simulink model "Ecuaciones_Fisicas_2020a"  (Simulink 10.1)
settings: Solver=FixedStepAuto  StartTime=0.0  StopTime=5  FixedStep=0.001  RelTol=1e-3
undefined symbols (not defined in the file or in its folder): magnitude, sigbuilder_block
libraries: simulink x2, simulink_extras x1
settings Model: Creator=alvar  LastModifiedBy=alvar  PauseTimes=2.78
settings DataIOCC: SaveFormat=Dataset  ReturnWorkspaceOutputs=on
settings OptimizationCC: LifeSpan=auto
settings DebuggingCC: UnderspecifiedInitializationDetection=Simplified  MergeDetectMultiDrivingBlocksExec=error  SFUnexpectedBacktrackingDiag=error  SFNoUnconditionalDefaultTransitionDiag=error  SFExecutionAtInitializationDiag=warning  ArithmeticOperatorsInVariantConditions=error
settings HardwareCC: ProdBitPerPointer=64  ProdBitPerSizeT=64  ProdBitPerPtrDiffT=64  ProdLargestAtomicFloat=Float  ProdIntDivRoundTo=Zero  ProdEndianess=LittleEndian  ProdWordSize=64  ProdHWDeviceType=Intel->x86-64 (Windows64)
settings ModelReferenceCC: PropagateSignalLabelsOutOfModel=on
settings SFSimCC: SimUseLocalCustomCode=on  CustomCodeUndefinedFunction=FilterOut
settings RTWCC: RTWUseLocalCustomCode=on
settings CodeAppCC: StateflowObjectComments=off
settings GRTTargetCC: TargetLangStandard=C99 (ISO)  CombineOutputUpdateFcns=on  GRTInterface=off
settings ConfigComp: CovMetricSettings=dwe  CovSaveCumulativeToWorkspaceVar=off  CovSaveSingleToWorkspaceVar=off  CovExternalEMLEnable=on

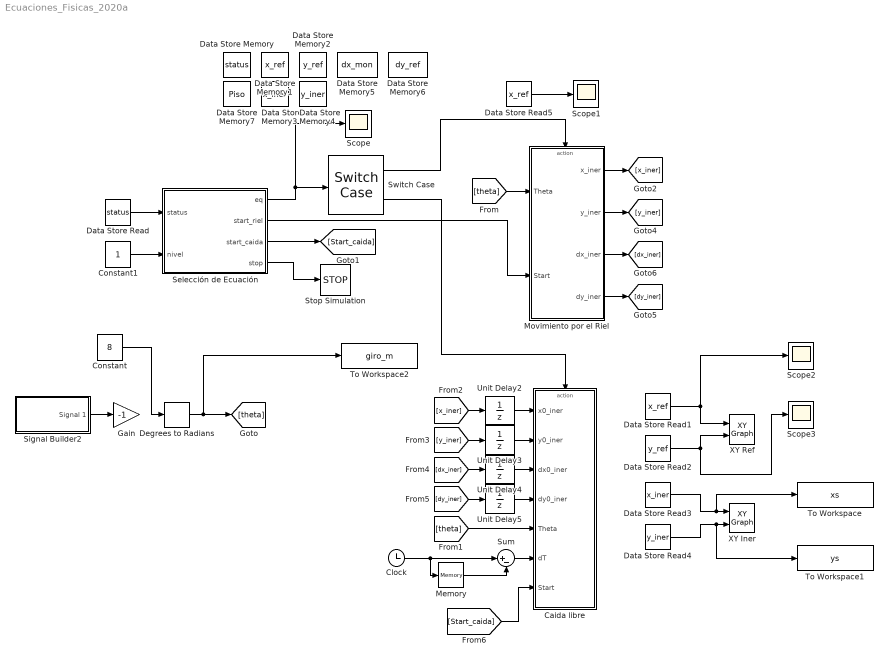
== system Ecuaciones_Fisicas_2020a ==
  Caida libre : Subsystem  TreatAsAtomicUnit=on
  Clock : Clock
  Constant : Constant  Value=8
  Constant1 : Constant
  Data Store Memory : DataStoreMemory  DataStoreName=status  ReadBeforeWriteMsg=warning  WriteAfterWriteMsg=warning  WriteAfterReadMsg=warning  ShowAdditionalParam=off  OutDataTypeStr=double
  Data Store Memory1 : DataStoreMemory  DataStoreName=x_ref  ReadBeforeWriteMsg=warning  WriteAfterWriteMsg=warning  WriteAfterReadMsg=warning  InitialValue=-0.11  ShowAdditionalParam=off  OutDataTypeStr=double
  Data Store Memory2 : DataStoreMemory  DataStoreName=y_ref  ReadBeforeWriteMsg=warning  WriteAfterWriteMsg=warning  WriteAfterReadMsg=warning  ShowAdditionalParam=off  OutDataTypeStr=double
  Data Store Memory3 : DataStoreMemory  DataStoreName=x_iner  ReadBeforeWriteMsg=warning  WriteAfterWriteMsg=warning  WriteAfterReadMsg=warning  InitialValue=-0.11  ShowAdditionalParam=off  OutDataTypeStr=double
  Data Store Memory4 : DataStoreMemory  DataStoreName=y_iner  ReadBeforeWriteMsg=warning  WriteAfterWriteMsg=warning  WriteAfterReadMsg=warning  ShowAdditionalParam=off  OutDataTypeStr=double
  Data Store Memory5 : DataStoreMemory  DataStoreName=dx_mon  ReadBeforeWriteMsg=warning  WriteAfterWriteMsg=warning  WriteAfterReadMsg=warning  ShowAdditionalParam=off  OutDataTypeStr=double
  Data Store Memory6 : DataStoreMemory  DataStoreName=dy_ref  ReadBeforeWriteMsg=warning  WriteAfterWriteMsg=warning  WriteAfterReadMsg=warning  ShowAdditionalParam=off  OutDataTypeStr=double
  Data Store Memory7 : DataStoreMemory  DataStoreName=Piso  ReadBeforeWriteMsg=warning  WriteAfterWriteMsg=warning  WriteAfterReadMsg=warning  InitialValue=1  ShowAdditionalParam=off  OutDataTypeStr=double
  Data Store Read : DataStoreRead  DataStoreName=status
  Data Store Read1 : DataStoreRead  DataStoreName=x_ref
  Data Store Read2 : DataStoreRead  DataStoreName=y_ref
  Data Store Read3 : DataStoreRead  DataStoreName=x_iner
  Data Store Read4 : DataStoreRead  DataStoreName=y_iner
  Data Store Read5 : DataStoreRead  DataStoreName=x_ref
  Degrees to Radians : simulink_extras/Transformations/Degrees to Radians
  Gain : Gain  Gain=-1
  Memory : Memory
  Movimiento por el Riel : Subsystem  TreatAsAtomicUnit=on
  Scope{,1..3} (4 alike) : Scope
  Selección de Ecuación : MATLAB Function  TreatAsAtomicUnit=on
  Signal Builder2 : Subsystem  Tag=STV Subsys  LoadFcn=sigbuilder_block('load');  StartFcn=sigbuilder_block('start');  StopFcn=sigbuilder_block('stop');  ClipboardFcn=sigbuilder_block('clipboard');  mask(Sigbuilder block){tuvar=[0:10]}
      mask help: Simulink:masks:SigbuilderBlock_MD
      mask init:
      | if ~strcmp(get_param(bdroot(gcbh),'SimulationStatus'),'stopped') tuvar = sigbuilder_block('maskInit'); end
      settings: CopyFcn=sigbuilder_block('copy');  DeleteFcn=sigbuilder_block('delete');  ModelCloseFcn=sigbuilder_block('modelClose');  PreSaveFcn=sigbuilder_block('preSave');  PauseFcn=sigbuilder_block('pause');  ContinueFcn=sigbuilder_block('continue');  NameChangeFcn=sigbuilder_block('namechange');  OpenFcn=sigbuilder_block('open',[516 235.5 550.5 399.75 ]);  CloseFcn=sigbuilder_block('close');
      mask Display: plot(0, 0, 100, 100,[2, 2, 32, 32, 2], [68, 8, 8, 68, 68],[32, 2], [38, 38], [32, 19, 2],[53, 60, 44], [32, 17, 17, 2],[16, 16, 31, 31]);txt = getActiveGroup(gcbh);text(2, 100, txt,'verticalAlignment', 'top');
  Stop Simulation : Stop
  Sum : Sum  Inputs=|+-
  Switch Case : SwitchCase  CaseConditions={1,2}  ShowDefaultCase=off
  To Workspace : ToWorkspace  VariableName=xs  SampleTime=0.01
  To Workspace1 : ToWorkspace  VariableName=ys  SampleTime=0.01
  To Workspace2 : ToWorkspace  VariableName=giro_m  SampleTime=0.01
  Unit Delay{2..5} (4 alike) : UnitDelay  SampleTime=-1  HasFrameUpgradeWarning=on
  XY Iner : simulink/Sinks/XY Graph  xmin=-0.15  xmax=0.15  ymin=-0.3  ymax=0.2  st=-1
  XY Ref : simulink/Sinks/XY Graph  xmin=-0.15  xmax=0.15  ymin=-0.3  ymax=0.2  st=-1
  wires:
  Switch Case/1 -> Movimiento por el Riel/Action
  [theta] -> Movimiento por el Riel/1(Theta)
  Switch Case/2 -> Caida libre/Action
  Selección de Ecuación/1(eq) -> Switch Case/1, Scope/1
  Data Store Read/1 -> Selección de Ecuación/1(status)
  Degrees to Radians/1 -> To Workspace2/1, [theta]
  Memory/1 -> Sum/2
  Clock/1 -> Sum/1, Memory/1
  Sum/1 -> Caida libre/6(dT)
  [x_iner] -> Unit Delay2/1
  Unit Delay2/1 -> Caida libre/1(x0_iner)
  [y_iner] -> Unit Delay3/1
  Unit Delay3/1 -> Caida libre/2(y0_iner)
  [dx_iner] -> Unit Delay4/1
  Unit Delay4/1 -> Caida libre/3(dx0_iner)
  [dy_iner] -> Unit Delay5/1
  Unit Delay5/1 -> Caida libre/4(dy0_iner)
  [theta] -> Caida libre/5(Theta)
  Data Store Read1/1 -> Scope2/1, XY Ref/1
  Data Store Read2/1 -> XY Ref/2, Scope3/1
  Data Store Read4/1 -> To Workspace1/1, XY Iner/2
  Data Store Read3/1 -> To Workspace/1, XY Iner/1
  Movimiento por el Riel/1(x_iner) -> [x_iner]
  Movimiento por el Riel/3(dx_iner) -> [dx_iner]
  Movimiento por el Riel/2(y_iner) -> [y_iner]
  Movimiento por el Riel/4(dy_iner) -> [dy_iner]
  Selección de Ecuación/2(start_riel) -> Movimiento por el Riel/2(Start)
  Signal Builder2/1(Signal 1) -> Gain/1
  Data Store Read5/1 -> Scope1/1
  Constant/1 -> Degrees to Radians/1
  Selección de Ecuación/3(start_caida) -> [Start_caida]
  [Start_caida] -> Caida libre/7(Start)
  Constant1/1 -> Selección de Ecuación/2(nivel)
  Selección de Ecuación/4(stop) -> Stop Simulation/1

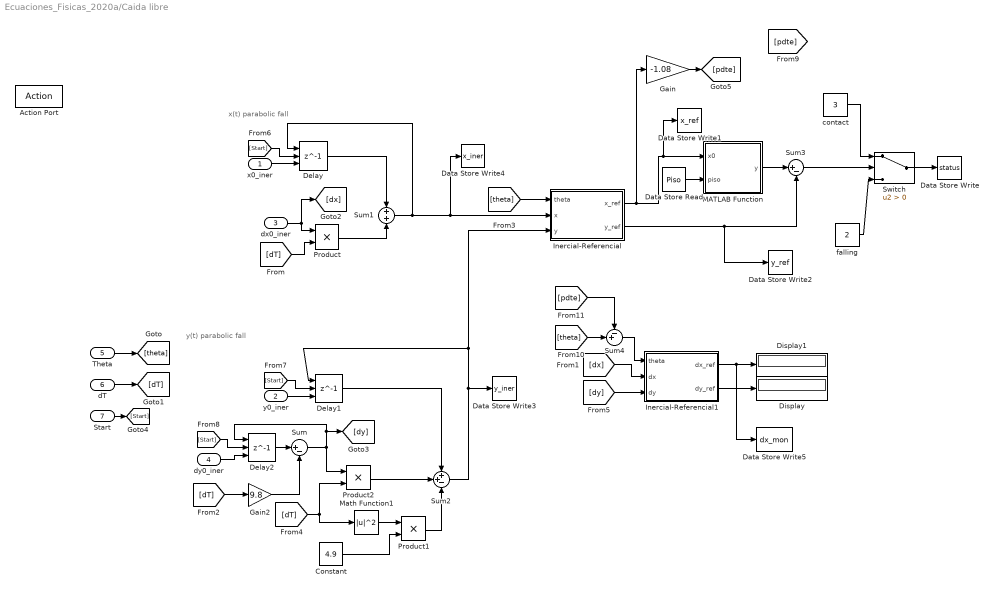
== system Ecuaciones_Fisicas_2020a/Caida libre ==
  note: x(t) parabolic fall
  note: y(t) parabolic fall
  x0_iner : Inport
  y0_iner : Inport  Port=2
  dx0_iner : Inport  Port=3
  dy0_iner : Inport  Port=4
  Theta : Inport  Port=5
  dT : Inport  Port=6
  Start : Inport  Port=7
  Action Port : ActionPort  ActionPortLabel=case [ 2 ]:
  Constant : Constant  Value=4.9
  Data Store Read : DataStoreRead  DataStoreName=Piso
  Data Store Write : DataStoreWrite  DataStoreName=status
  Data Store Write1 : DataStoreWrite  DataStoreName=x_ref
  Data Store Write2 : DataStoreWrite  DataStoreName=y_ref
  Data Store Write3 : DataStoreWrite  DataStoreName=y_iner
  Data Store Write4 : DataStoreWrite  DataStoreName=x_iner
  Data Store Write5 : DataStoreWrite  DataStoreName=dx_mon
  Delay : Delay  DelayLength=1  InitialConditionSource=Input port  ExternalReset=Rising
      settings: InputPortMap=u0,r5,p4
  Delay1 : Delay  DelayLength=1  InitialConditionSource=Input port  ExternalReset=Rising
      settings: InputPortMap=u0,r5,p4
  Delay2 : Delay  DelayLength=1  InitialConditionSource=Input port  ExternalReset=Rising
      settings: InputPortMap=u0,r5,p4
  Display : Display
  Display1 : Display
  Gain : Gain  Gain=-1.08
  Gain2 : Gain  Gain=9.8
  Inercial-Referencial : MATLAB Function  TreatAsAtomicUnit=on
  Inercial-Referencial1 : MATLAB Function  TreatAsAtomicUnit=on
  MATLAB Function : MATLAB Function  TreatAsAtomicUnit=on
  Math Function1 : Math  Operator=magnitude^2  SaturateOnIntegerOverflow=on
  Product : Product
  Product1 : Product
  Product2 : Product
  Sum : Sum  Inputs=|+-
  Sum1 : Sum
  Sum2 : Sum  Inputs=++-
  Sum3 : Sum  Inputs=|+-
  Sum4 : Sum  Inputs=-+|
  Switch : Switch  Criteria=u2 > Threshold
  contact : Constant  Value=3
  falling : Constant  Value=2
  wires:
  [dT] -> Product/2
  Product/1 -> Sum1/2
  Delay1/1 -> Sum2/1
  [dT] -> Math Function1/1, Product2/2
  Sum1/1 -> Data Store Write4/1, Inercial-Referencial/2(x), Delay/1
  Product2/1 -> Sum2/2
  Product1/1 -> Sum2/3
  Math Function1/1 -> Product1/1
  Theta/1 -> [theta]
  x0_iner/1 -> Delay/3
  Delay/1 -> Sum1/1
  dT/1 -> [dT]
  dx0_iner/1 -> [dx], Product/1
  y0_iner/1 -> Delay1/3
  Sum2/1 -> Inercial-Referencial/3(y), Delay1/1, Data Store Write3/1
  dy0_iner/1 -> Delay2/3
  Delay2/1 -> Sum/1
  [dT] -> Gain2/1
  Gain2/1 -> Sum/2
  Sum/1 -> Product2/1, [dy], Delay2/1
  [theta] -> Inercial-Referencial/1(theta)
  Constant/1 -> Product1/2
  [dx] -> Inercial-Referencial1/2(dx)
  [dy] -> Inercial-Referencial1/3(dy)
  Inercial-Referencial/1(x_ref) -> Gain/1, Data Store Write1/1, MATLAB Function/1(x0)
  Data Store Read/1 -> MATLAB Function/2(piso)
  MATLAB Function/1(y) -> Sum3/1
  Inercial-Referencial/2(y_ref) -> Data Store Write2/1, Sum3/2
  falling/1 -> Switch/3
  Sum3/1 -> Switch/2
  Switch/1 -> Data Store Write/1
  contact/1 -> Switch/1
  Inercial-Referencial1/1(dx_ref) -> Data Store Write5/1, Display1/1
  Inercial-Referencial1/2(dy_ref) -> Display/1
  Start/1 -> [Start]
  [Start] -> Delay/2
  [Start] -> Delay1/2
  [Start] -> Delay2/2
  Gain/1 -> [pdte]
  [theta] -> Sum4/2
  [pdte] -> Sum4/1
  Sum4/1 -> Inercial-Referencial1/1(theta)

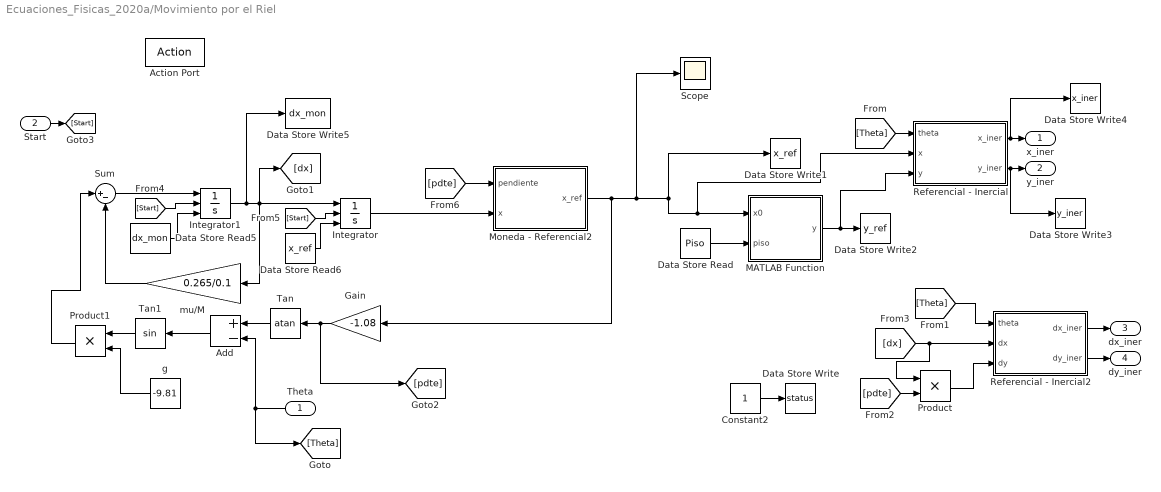
== system Ecuaciones_Fisicas_2020a/Movimiento por el Riel ==
  Theta : Inport
  Start : Inport  Port=2
  Action Port : ActionPort  ActionPortLabel=case [ 1 ]:
  Add : Sum  Inputs=+-
  Constant2 : Constant
  Data Store Read : DataStoreRead  DataStoreName=Piso
  Data Store Read5 : DataStoreRead  DataStoreName=dx_mon
  Data Store Read6 : DataStoreRead  DataStoreName=x_ref
  Data Store Write : DataStoreWrite  DataStoreName=status
  Data Store Write1 : DataStoreWrite  DataStoreName=x_ref
  Data Store Write2 : DataStoreWrite  DataStoreName=y_ref
  Data Store Write3 : DataStoreWrite  DataStoreName=y_iner
  Data Store Write4 : DataStoreWrite  DataStoreName=x_iner
  Data Store Write5 : DataStoreWrite  DataStoreName=dx_mon
  Gain : Gain  Gain=-1.08
  Integrator : Integrator  ExternalReset=rising  InitialConditionSource=external
  Integrator1 : Integrator  ExternalReset=rising  InitialConditionSource=external
  MATLAB Function : MATLAB Function  TreatAsAtomicUnit=on
  Moneda - Referencial2 : MATLAB Function  TreatAsAtomicUnit=on
  Product : Product
  Product1 : Product
  Referencial - Inercial : MATLAB Function  TreatAsAtomicUnit=on
  Referencial - Inercial2 : MATLAB Function  TreatAsAtomicUnit=on
  Scope : Scope
  Sum : Sum  Inputs=|+-
  Tan : Trigonometry  Operator=atan
  Tan1 : Trigonometry
  g : Constant  Value=-9.81
  mu/M : Gain  Gain=0.265/0.1
  x_iner : Outport
  y_iner : Outport  Port=2
  dx_iner : Outport  Port=3
  dy_iner : Outport  Port=4
  wires:
  Add/1 -> Tan1/1
  Tan/1 -> Add/1
  Gain/1 -> [pdte], Tan/1
  mu/M/1 -> Sum/2
  g/1 -> Product1/2
  Integrator1/1 -> Data Store Write5/1, [dx], mu/M/1, Integrator/1
  Data Store Read5/1 -> Integrator1/3
  Sum/1 -> Integrator1/1
  Tan1/1 -> Product1/1
  Data Store Read6/1 -> Integrator/3
  Theta/1 -> [Theta], Add/2
  Data Store Read/1 -> MATLAB Function/2(piso)
  MATLAB Function/1(y) -> Data Store Write2/1, Referencial - Inercial/3(y)
  Constant2/1 -> Data Store Write/1
  Referencial - Inercial/1(x_iner) -> Data Store Write4/1, x_iner/1
  Referencial - Inercial/2(y_iner) -> Data Store Write3/1, y_iner/1
  [Theta] -> Referencial - Inercial/1(theta)
  [Theta] -> Referencial - Inercial2/1(theta)
  Referencial - Inercial2/2(dy_iner) -> dy_iner/1
  Referencial - Inercial2/1(dx_iner) -> dx_iner/1
  [dx] -> Product/1, Referencial - Inercial2/2(dx)
  Product/1 -> Referencial - Inercial2/3(dy)
  [pdte] -> Product/2
  Start/1 -> [Start]
  [Start] -> Integrator1/2
  [Start] -> Integrator/2
  Integrator/1 -> Moneda - Referencial2/2(x)
  Moneda - Referencial2/1(x_ref) -> Gain/1, Scope/1, Data Store Write1/1, Referencial - Inercial/2(x), MATLAB Function/1(x0)
  [pdte] -> Moneda - Referencial2/1(pendiente)
  Product1/1 -> Sum/1

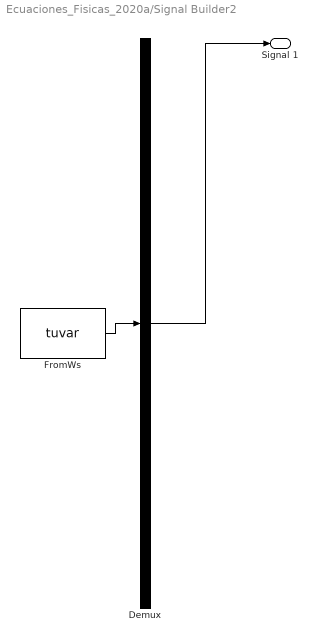
== system Ecuaciones_Fisicas_2020a/Signal Builder2 ==
  Demux : Demux  Tag=STV Demux  Outputs=1
      settings: DisplayOption=none
  FromWs : FromWorkspace  Tag=STV FromWs  VariableName=tuvar  SigBuilderData=DataTag0  VnvData=DataTag1
      SigBuilderData=|
      | common.afterFinalStr = 'Extrapolate'
      | common.sampleTime = 0
      | dataSet.timeRange = [0 20]
      | dataSet.name = 'Group 1'
      | sbobj.Groups.Name = 'Group 1'
      | sbobj.Groups.Signals.Name = 'Signal 1'
      | sbobj.Groups.Signals.XData = [0 1.75 1.76 2.443 2.45 3.6 3.835 3.84 4.5 4.984 4.99 5.8 6.2 6.3 6.5 6.51 20]
      | sbobj.Groups.Signals.YData = [-7 -7 15 15 -15 -10 -10 15 7.5 7.5 -15 -10.4 -7 5 5 12 12]
      | sbobj.Groups.TimeRange = [0 20]
  Signal 1 : Outport  Tag=STV Outport
  wires:
  Demux/1 -> Signal 1/1
  FromWs/1 -> Demux/1

== matlab function Movimiento por el Riel/Moneda - Referencial2 ==
  settings: updateMethod=DISCRETE
  data: pendiente input double; x_ref output double; x input double
function x_ref  = rotate(pendiente,x)
x_ref =  x*cos(-pendiente);

== matlab function Movimiento por el Riel/MATLAB Function ==
  data: x0 input double; y output double; piso input double
function y  = fcn(x0, piso)

switch piso
    case 1
        y= -0.54*x0^2 + 0.1143;
    case 2
        y= -0.54*x0^2 + 0.0686;
    case 3
        y= -0.54*x0^2 + 0.03;
    case 4
        y= -0.54*x0^2 - 0.03;  
    case 5
        y= -0.54*x0^2 - 0.0686; 
    case 6
        y= -0.54*x0^2 - 0.1143;
    case 7
        y= -0.54*x0^2 - 0.16;
    otherwise
        y = 0;
end

== matlab function Caida libre/Inercial-Referencial ==
  settings: updateMethod=DISCRETE
  data: theta input double; x_ref output double; x input double; y input double; y_ref output double
function [x_ref,y_ref] = rotate(theta,x,y)
x_ref = x*cos(theta) - y*sin(theta);
y_ref = x*sin(theta) + y*cos(theta);

== matlab function Selección de Ecuación ==
  settings: updateMethod=DISCRETE
  data: eq output double; status input double; x_ref data_store_memory double; Piso data_store_memory double; start_riel output double; start_caida output double; stop output double; nivel input double
function [eq, start_riel, start_caida, stop] = fcn(status, nivel)

%%DE MOMENTO ESTE CÓDIGO ES PARA PROBAR LAS ECUACIONES EN LA PRIMERA CAIDA
persistent x_edges
persistent equation
global x_ref;
global Piso;
start_riel = 0;
start_caida = 0;
stop = 0;
if(isempty(equation))
    equation = 1;
end
coder.extrinsic('fallCoor');
if (isempty(x_edges))
    x_edges = zeros(7,2);
    x_edges = fallCoor(nivel);
end
%x_edges = fallCoor(1)

if(status == 1)
    switch Piso
        case 1
            if (x_ref > x_edges(1,1)) %starts falling
              equation = 2;
              start_caida = 1;
            elseif (x_ref < x_edges(1,2))
                stop = 1;
            end
            
        case 2
            if (x_ref < x_edges(2,2))
                equation = 2;
                start_caida = 1;
            elseif (x_ref > x_edges(2,1))
                stop = 1;
                disp('Caida Piso1');
            end
        case 3
            if (x_ref > x_edges(3,1))
                equation = 2;
                start_caida = 1;
            elseif (x_ref < x_edges(3,2))
                stop = 1;
            end
        case 4
            if (x_ref < x_edges(4,2))
                equation = 2;
                start_caida = 1;
            elseif (x_ref > x_edges(4,1))
                stop = 1;
            end
        case 5
            if (x_ref > x_edges(5,1))
                equation = 2;
                start_caida = 1;
            elseif (x_ref < x_edges(5,2))
                stop = 1;
            end
        case 6
            if (x_ref < x_edges(6,2))
                equation = 2;
                start_caida = 1;
            elseif (x_ref > x_edges(6,1))
                stop = 1;
            end
        case 7
            if (x_ref > x_edges(7,1))
                equation = 2;
                start_caida = 1;
            elseif (x_ref < x_edges(7,2))
                stop = 1;
            end
    end
end

if(status == 3) %impact
    equation = 1;
    Piso = Piso + 1;
    start_riel = 1;
end

eq = equation;

== matlab function Caida libre/Inercial-Referencial1 ==
  settings: updateMethod=DISCRETE
  data: theta input double; dx_ref output double; dx input double; dy input double; dy_ref output double
function [dx_ref,dy_ref] = rotate(theta,dx,dy)
dx_ref = dx*cos(theta) - dy*sin(theta);
dy_ref = dx*sin(theta) + dy*cos(theta);

== matlab function Caida libre/MATLAB Function ==
  data: x0 input double; y output double; piso input double
function y  = fcn(x0, piso)

paux = piso+1;
switch paux
    case 1
        y= -0.54*x0^2 + 0.1143;
    case 2
        y= -0.54*x0^2 + 0.0686;
    case 3
        y= -0.54*x0^2 + 0.03;
    case 4
        y= -0.54*x0^2 - 0.03;
    case 5
        y= -0.54*x0^2 - 0.0686; 
    case 6
        y= -0.54*x0^2 - 0.1143;
    case 7
        y= -0.54*x0^2 - 0.16;
    otherwise
        y = 0;
end

== matlab function Movimiento por el Riel/Referencial - Inercial ==
  settings: updateMethod=DISCRETE
  data: theta input double; x_iner output double; x input double; y input double; y_iner output double
function [x_iner,y_iner] = rotate(theta,x,y)
x_iner =  x*cos(theta) + y*sin(theta);
y_iner = -x*sin(theta) + y*cos(theta);

== matlab function Movimiento por el Riel/Referencial - Inercial2 ==
  settings: updateMethod=DISCRETE
  data: theta input double; dx_iner output double; dx input double; dy input double; dy_iner output double
function [dx_iner,dy_iner] = rotate(theta,dx,dy)
dx_iner =  dx*cos(-theta) - dy*sin(-theta);
dy_iner = dx*sin(-theta) + dy*cos(-theta);
